simulink model "GovModel"  (R2014a)
settings: Solver=ode3  StartTime=tstart  StopTime=tstop  FixedStep=dt  RelTol=1e-3
values from neighbouring files (symbols this model uses):
  Dt = 0    [SimulinkGov.m]
  R = 0.05    [SimulinkGov.m]
  T1 = 0.5    [SimulinkGov.m]
  T2 = 3.0    (= 3)    [SimulinkGov.m]
  T3 = 10    [SimulinkGov.m]
settings Model: Creator=mstajcar  LastModifiedBy=MStajcar

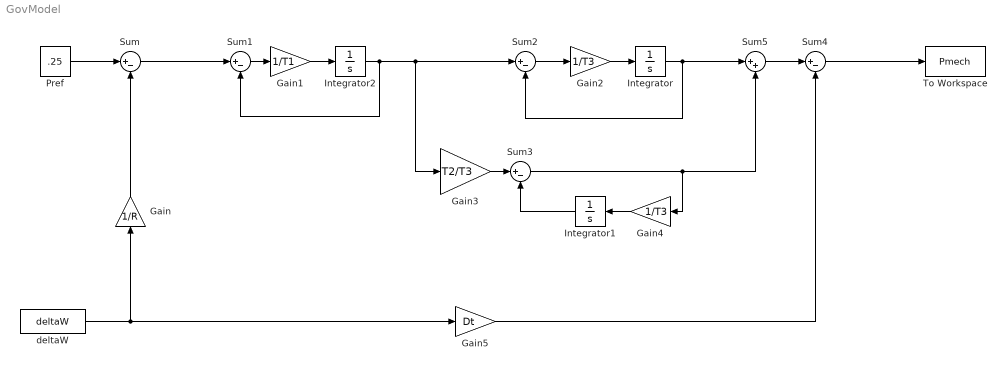
== system GovModel ==
  Gain : Gain  Gain=1/R
  Gain1 : Gain  Gain=1/T1
  Gain2 : Gain  Gain=1/T3
  Gain3 : Gain  Gain=T2/T3
  Gain4 : Gain  Gain=1/T3
  Gain5 : Gain  Gain=Dt
  Integrator : Integrator
  Integrator1 : Integrator
  Integrator2 : Integrator
  Pref : Constant  Value=.25
  Sum{,1..4} (5 alike) : Sum  Inputs=|+-
  Sum5 : Sum  Inputs=|++
  To Workspace : ToWorkspace  VariableName=Pmech  SampleTime=-1
  deltaW : FromWorkspace  VariableName=deltaW  SampleTime=0
  wires:
  Sum/1 -> Sum1/1
  Sum1/1 -> Gain1/1
  Gain1/1 -> Integrator2/1
  Sum2/1 -> Gain2/1
  Gain2/1 -> Integrator/1
  Integrator/1 -> Sum5/1, Sum2/2
  Gain3/1 -> Sum3/1
  Sum4/1 -> To Workspace/1
  Sum3/1 -> Gain4/1, Sum5/2
  Integrator1/1 -> Sum3/2
  Gain4/1 -> Integrator1/1
  Gain5/1 -> Sum4/2
  deltaW/1 -> Gain/1, Gain5/1
  Pref/1 -> Sum/1
  Integrator2/1 -> Gain3/1, Sum2/1, Sum1/2
  Sum5/1 -> Sum4/1
  Gain/1 -> Sum/2
